simulink model "sf_gfrecursive"  (Simulink 6.0)
settings: Solver=ode5  StartTime=0.0  StopTime=1  FixedStep=1  RelTol=1e-3
settings Model: CovMetricSettings=dcmtr  Creator=The MathWorks Inc.  LastModifiedBy=batserve  ExtModeAutoUpdateStatusClock=off
settings OptimizationCC: BooleanDataType=off
settings DebuggingCC: CheckExecutionContextPreStartOutputMsg=on  CheckExecutionContextRuntimeOutputMsg=on  SolverPrmCheckMsg=none
settings HardwareCC: TargetUnknown=on

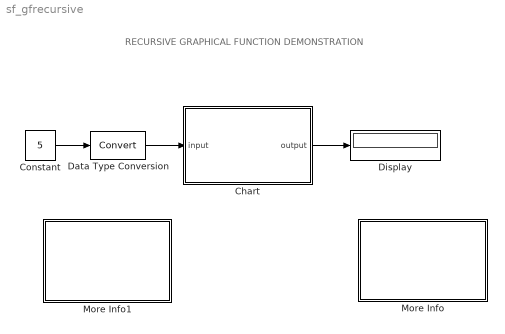
== system sf_gfrecursive ==
  note: RECURSIVE GRAPHICAL FUNCTION DEMONSTRATION
  Chart : Stateflow chart  PropExecContextAcrossSSBoundary=on
  Constant : Constant  Value=5
  Data Type Conversion : DataTypeConversion  OutDataTypeMode=uint32  SaturateOnIntegerOverflow=on  RndMeth=Zero
  Display : Display
  More Info : Subsystem  PropExecContextAcrossSSBoundary=on
      mask Display: disp('Double click\nhere for\ninformation on\nthis demonstration')
  More Info1 : Subsystem  PropExecContextAcrossSSBoundary=on
      settings: OpenFcn=simcad(bdroot);
      mask Display: disp('Double click\nhere for\nSimulink\Stateflow\n Help')
  wires:
  Chart/1(output) -> Display/1
  Constant/1 -> Data Type Conversion/1
  Data Type Conversion/1 -> Chart/1(input)

== system sf_gfrecursive/More Info ==
  note: RECURSIVE GRAPHICAL FUNCTION DEMONSTRATION
  note: This demonstration illustrates how graphical functions can be used as recursive functions.
      | The graphical function in the chart (called FACTORIAL) returns the factorial value of the input.
      | This is possible because graphical functions can be called from within themselves or from within
      |  other graphical functions. The risk in using a recursive function, is the possibility of creating an
      | infinite loop. In this example, FACTORIAL is called when the input value satisfies a certain condition.
      | If the condition is not satisfied, another path within the function is taken and the output in this path
      | is not dependent on the FACTORIAL function.

== system sf_gfrecursive/More Info1 ==

== stateflow chart Chart ==
  state result = factorial(n) [function]
    (junction 5) -> (junction 4) : [n==0]{result = 1;}
    (default) -> (junction 5)
    (junction 5) -> (junction 4) : [n>0 && n<21]
        | {result = n*factorial(n-1);}
    (junction 5) -> (junction 4) : /* if n >21, abort */
        | {result = 0;}
  (default) -> (junction 6) : {output = factorial(input);}
  data: n function_input uint32; result function_output uint32; input input uint32; output output uint32
